simulink model "stopwatch_th"  (R2018b)
settings: Solver=FixedStepDiscrete  StartTime=0.0  StopTime=10.0  FixedStep=0.001  RelTol=1e-3
libraries: simulink x1, stopwatch_ul x1
settings Model: Creator=mcobb  LastModifiedBy=mcobb

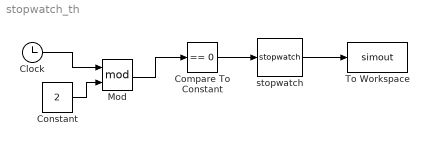
== system stopwatch_th ==
  Clock : Clock
  Compare To Constant : simulink/Logic and Bit Operations/Compare To Constant  relop===  const=0  OutDataTypeStr=boolean
  Constant : Constant  Value=2
  Mod : Math  Operator=mod  SaturateOnIntegerOverflow=on
  To Workspace : ToWorkspace  VariableName=simout  SaveFormat=Timeseries  SampleTime=-1
  stopwatch : stopwatch_ul/stopwatch  SystemSampleTime=-1
  wires:
  Clock/1 -> Mod/1
  Constant/1 -> Mod/2
  Mod/1 -> Compare To Constant/1
  Compare To Constant/1 -> stopwatch/1
  stopwatch/1 -> To Workspace/1
